simulink library "data_driven_lib_ctl"  (R2024a)
settings: Solver=VariableStepAuto  StartTime=0.0  StopTime=10.0  RelTol=1e-3
undefined symbols (not defined in the file or in its folder): ATDeePC_data, ATDeePC_DT, ATDeePC_LT, ATDeePC_params, ATDeePC_PT, ATDeePC_trajectory_T, ATDeePC_tune_data, ATDeePC_tune_DT, ATDeePC_tune_input_T, ATDeePC_tune_LT, ATDeePC_tune_params, ATDeePC_tune_PT, ATDeePC_tune_trajectory_T, DeePC_data, DeePC_DT, DeePC_LT, DeePC_params, DeePC_PT, DeePCPI_data, DeePCPI_DT, DeePCPI_LT, DeePCPI_params, DeePCPI_PT, extrinsic
settings Model: Creator=luka  LastModifiedBy=luka

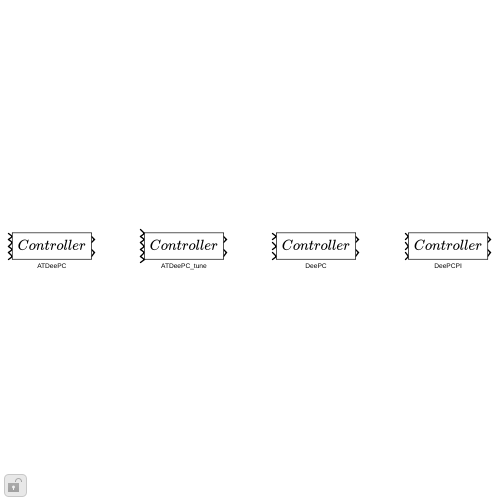
[thumbnail: Simulink's stored preview of the top-level diagram]
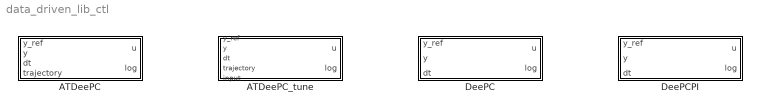
== system data_driven_lib_ctl ==
  ATDeePC : Subsystem  Tag=__cs_m_ctl;  mask{params=ATDeePC_params, data=ATDeePC_data, ParamsType=ATDeePC_PT, DataType=ATDeePC_DT, LogEntryType=ATDeePC_LT, u_ic=0, trajectory_T=ATDeePC_trajectory_T}
      mask prompts: params "Parameter struct:"
  ATDeePC_tune : Subsystem  Tag=__cs_m_ctl;  mask{params=ATDeePC_tune_params, data=ATDeePC_tune_data, ParamsType=ATDeePC_tune_PT, DataType=ATDeePC_tune_DT, LogEntryType=ATDeePC_tune_LT, u_ic=0, trajectory_T=ATDeePC_tune_trajectory_T, input_T=ATDeePC_tune_input_T}
      mask prompts: params "Parameter struct:"
  DeePC : Subsystem  Tag=__cs_m_ctl;  mask{params=DeePC_params, data=DeePC_data, ParamsType=DeePC_PT, DataType=DeePC_DT, LogEntryType=DeePC_LT, u_ic=0}
      mask prompts: params "Parameter struct:"
  DeePCPI : Subsystem  Tag=__cs_m_ctl;  mask{params=DeePCPI_params, data=DeePCPI_data, ParamsType=DeePCPI_PT, DataType=DeePCPI_DT, LogEntryType=DeePCPI_LT, u_ic=0}
      mask prompts: params "Parameter struct:"

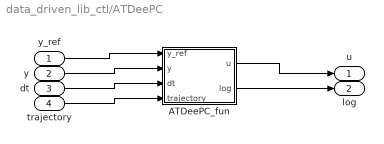
== system data_driven_lib_ctl/ATDeePC ==
  y_ref : Inport
  y : Inport  Port=2
  dt : Inport  Port=3
  trajectory : Inport  Port=4
  ATDeePC_fun : MATLAB Function  TreatAsAtomicUnit=on
  u : Outport
  log : Outport  Port=2
  wires:
  y_ref/1 -> ATDeePC_fun/1(y_ref)
  y/1 -> ATDeePC_fun/2(y)
  dt/1 -> ATDeePC_fun/3(dt)
  trajectory/1 -> ATDeePC_fun/4(trajectory)
  ATDeePC_fun/1(u) -> u/1
  ATDeePC_fun/2(log) -> log/1

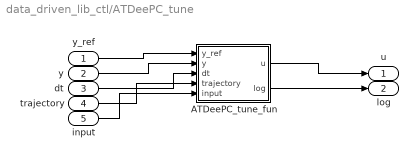
== system data_driven_lib_ctl/ATDeePC_tune ==
  y_ref : Inport
  y : Inport  Port=2
  dt : Inport  Port=3
  trajectory : Inport  Port=4
  input : Inport  Port=5
  ATDeePC_tune_fun : MATLAB Function  TreatAsAtomicUnit=on
  u : Outport
  log : Outport  Port=2
  wires:
  y_ref/1 -> ATDeePC_tune_fun/1(y_ref)
  y/1 -> ATDeePC_tune_fun/2(y)
  dt/1 -> ATDeePC_tune_fun/3(dt)
  trajectory/1 -> ATDeePC_tune_fun/4(trajectory)
  input/1 -> ATDeePC_tune_fun/5(input)
  ATDeePC_tune_fun/1(u) -> u/1
  ATDeePC_tune_fun/2(log) -> log/1

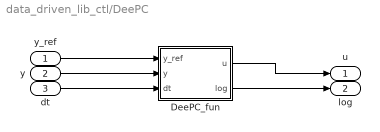
== system data_driven_lib_ctl/DeePC ==
  y_ref : Inport
  y : Inport  Port=2
  dt : Inport  Port=3
  DeePC_fun : MATLAB Function  TreatAsAtomicUnit=on
  u : Outport
  log : Outport  Port=2
  wires:
  y_ref/1 -> DeePC_fun/1(y_ref)
  y/1 -> DeePC_fun/2(y)
  dt/1 -> DeePC_fun/3(dt)
  DeePC_fun/1(u) -> u/1
  DeePC_fun/2(log) -> log/1

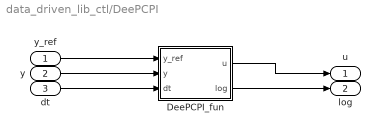
== system data_driven_lib_ctl/DeePCPI ==
  y_ref : Inport
  y : Inport  Port=2
  dt : Inport  Port=3
  DeePCPI_fun : MATLAB Function  TreatAsAtomicUnit=on
  u : Outport
  log : Outport  Port=2
  wires:
  y_ref/1 -> DeePCPI_fun/1(y_ref)
  y/1 -> DeePCPI_fun/2(y)
  dt/1 -> DeePCPI_fun/3(dt)
  DeePCPI_fun/1(u) -> u/1
  DeePCPI_fun/2(log) -> log/1

== matlab function data_driven_lib_ctl/ATDeePC_tune/ATDeePC_tune_fun ==
  settings: updateMethod=DISCRETE
  data: y_ref input; u output; y input; dt input; trajectory input trajectory_T; input input input_T; log output LogEntryType; extrinsic parameter int32; data parameter DataType; params parameter ParamsType; u_ic parameter double
% __classname:=ATDeePC_tune;
function [u, log] = fcn(y_ref, y, dt, trajectory, input, extrinsic, data, params, u_ic)
  coder.extrinsic('fcn_cc2ebf65f69845dcb8e3bf654c56ed7a_ext');
  if extrinsic
      u = u_ic;
      [u, log] = fcn_cc2ebf65f69845dcb8e3bf654c56ed7a_ext(y_ref, y, dt, trajectory, input, u_ic, params, data);
  else
      [u, log] = fcn_cc2ebf65f69845dcb8e3bf654c56ed7a(y_ref, y, dt, trajectory, input, u_ic, params, data);
  end
end

function [u, log] = fcn_cc2ebf65f69845dcb8e3bf654c56ed7a(y_ref, y, dt, trajectory, input, u_ic, params, data)
  persistent obj
  if isempty(obj)
    obj = ATDeePC_tune(params, 'Data', data);
    obj = obj.configure(1, size(y), size(y_ref));
  end
  [obj, u, log] = obj.step(y_ref, y, dt, trajectory, input);
end

== matlab function data_driven_lib_ctl/ATDeePC/ATDeePC_fun ==
  settings: updateMethod=DISCRETE
  data: y_ref input; u output; y input; dt input; trajectory input trajectory_T; log output LogEntryType; extrinsic parameter int32; data parameter DataType; params parameter ParamsType; u_ic parameter double
% __classname:=ATDeePC;
function [u, log] = fcn(y_ref, y, dt, trajectory, extrinsic, data, params, u_ic)
  coder.extrinsic('fcn_a76475e45c1141e1a5ad1ab93265023c_ext');
  if extrinsic
      u = u_ic;
      [u, log] = fcn_a76475e45c1141e1a5ad1ab93265023c_ext(y_ref, y, dt, trajectory, u_ic, params, data);
  else
      [u, log] = fcn_a76475e45c1141e1a5ad1ab93265023c(y_ref, y, dt, trajectory, u_ic, params, data);
  end
end

function [u, log] = fcn_a76475e45c1141e1a5ad1ab93265023c(y_ref, y, dt, trajectory, u_ic, params, data)
  persistent obj
  if isempty(obj)
    obj = ATDeePC(params, 'Data', data);
    obj = obj.configure(1, size(y), size(y_ref));
  end
  [obj, u, log] = obj.step(y_ref, y, dt, trajectory);
end

== matlab function data_driven_lib_ctl/DeePC/DeePC_fun ==
  settings: updateMethod=DISCRETE
  data: y_ref input; u output; y input; dt input; log output LogEntryType; extrinsic parameter int32; data parameter DataType; params parameter ParamsType; u_ic parameter double
% __classname:=DeePC;
function [u, log] = fcn(y_ref, y, dt, extrinsic, data, params, u_ic)
  coder.extrinsic('fcn_a2401829f74147a5abec788c567140ea_ext');
  if extrinsic
      u = u_ic;
      [u, log] = fcn_a2401829f74147a5abec788c567140ea_ext(y_ref, y, dt, u_ic, params, data);
  else
      [u, log] = fcn_a2401829f74147a5abec788c567140ea(y_ref, y, dt, u_ic, params, data);
  end
end

function [u, log] = fcn_a2401829f74147a5abec788c567140ea(y_ref, y, dt, u_ic, params, data)
  persistent obj
  if isempty(obj)
    obj = DeePC(params, 'Data', data);
    obj = obj.configure(1, size(y), size(y_ref));
  end
  [obj, u, log] = obj.step(y_ref, y, dt);
end

== matlab function data_driven_lib_ctl/DeePCPI/DeePCPI_fun ==
  settings: updateMethod=DISCRETE
  data: y_ref input; u output; y input; dt input; log output LogEntryType; extrinsic parameter int32; data parameter DataType; params parameter ParamsType; u_ic parameter double
% __classname:=DeePCPI;
function [u, log] = fcn(y_ref, y, dt, extrinsic, data, params, u_ic)
  coder.extrinsic('fcn_3d0611914e98445f9f19ad7f55c5f84b_ext');
  if extrinsic
      u = u_ic;
      [u, log] = fcn_3d0611914e98445f9f19ad7f55c5f84b_ext(y_ref, y, dt, u_ic, params, data);
  else
      [u, log] = fcn_3d0611914e98445f9f19ad7f55c5f84b(y_ref, y, dt, u_ic, params, data);
  end
end

function [u, log] = fcn_3d0611914e98445f9f19ad7f55c5f84b(y_ref, y, dt, u_ic, params, data)
  persistent obj
  if isempty(obj)
    obj = DeePCPI(params, 'Data', data);
    obj = obj.configure(1, size(y), size(y_ref));
  end
  [obj, u, log] = obj.step(y_ref, y, dt);
end
